simulink model "QAM_RX"  (R2018a)
settings: Solver=ode45  StartTime=0.0  StopTime=inf  RelTol=1e-3  EnableMultiTasking=on
values from neighbouring files (symbols this model uses):
  FrameTime = 0.000552    [qpsktxrx16.mat]
  qpsktxrx =     [qpsktxrx16.mat]
undefined symbols (not defined in the file or in its folder): dfilt, j
libraries: simulink x6, dspstat3 x6, dspobslib x6, dspsigops x5, commdigbbndam3 x4, commblkintrlv2 x4, commutil2 x4, commrflib2 x3, commblksprivate x2, dspspect3 x2, dspsrcs4 x2, commsink2 x2
(part 1 of 2)
settings Model: SimulationMode=accelerator  Creator=root  LastModifiedBy=n53s123
settings DataIOCC: LimitDataPoints=on  SaveFormat=Array
settings OptimizationCC: LifeSpan=inf
settings DebuggingCC: SolverPrmCheckMsg=warning  SFUnexpectedBacktrackingDiag=warning  SFNoUnconditionalDefaultTransitionDiag=warning  SFExecutionAtInitializationDiag=none
settings HardwareCC: ProdBitPerPointer=32  ProdBitPerSizeT=32  ProdBitPerPtrDiffT=32  ProdLargestAtomicFloat=None  ProdIntDivRoundTo=Undefined  ProdEndianess=Unspecified  ProdWordSize=32  ProdHWDeviceType=32-bit Generic
settings ModelReferenceCC: PropagateSignalLabelsOutOfModel=off
settings CodeAppCC: StateflowObjectComments=on
settings GRTTargetCC: TargetLangStandard=C89/C90 (ANSI)  GeneratePreprocessorConditionals=Disable all
settings ConfigComp: CovMetricSettings=dw  CovHtmlReporting=on  CovSaveCumulativeToWorkspaceVar=on  CovSaveSingleToWorkspaceVar=on  CovExternalEMLEnable=off  CovSFcnEnable=off

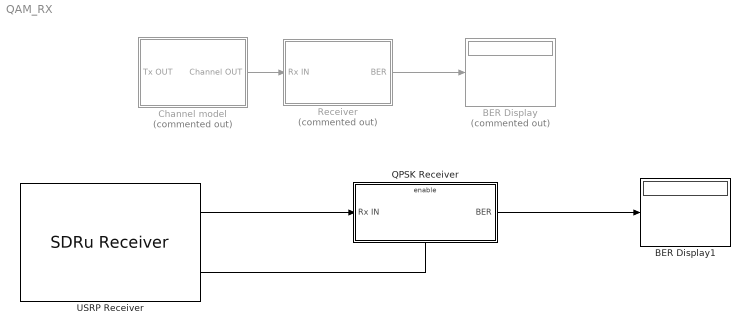
== system QAM_RX ==
  BER Display : Display  Commented=on
  BER Display1 : Display
  Channel model : Subsystem  Commented=on
  QPSK Receiver : Subsystem
      mask Display: disp('QAM Receiver')
  Receiver : Subsystem  Commented=on
      mask Display: disp('Receiver')
  USRP Receiver : commsdrhw_v2/SDRu Receiver  SourceLibraryInfo="This block requires <a href=\"http://www.mathworks.com/hardware-support/usrp.html\">Communications System Toolbox Support Package for USRP Radio</a>"  rxtx=rx  initializeIPAddress=0  devMap=0  USRP2_IP=192.168.10.2  USRP_IP_X300=192.168.10.2  USRP_IP_X310=192.168.10.2  USRP_serialNumB200=30B2ACA  USRP_serialNumB210=ECR04ZDBT  platform=N200/N210/USRP2  prevPlatform=N200/N210/USRP2  lastIPAddressPopup=192.168.10.2  USRP_ID=192.168.10.2  LastIPAddress=192.168.10.2  ChannelMapping=1  centerFrequencySrc=Dialog  centerFrequency=2.5e6  loOffsetSrc=Dialog  loOffset=0  gainSrc=Dialog  gain=0  PPSSource=Internal  clockSource=Internal  masterClkRateParam=100e6  masterClkRateB200=sdrqpskrx.MasterClockRate  masterClkRateB210=sdrqpskrx.MasterClockRate  masterClkRateX300=200e6  masterClkRateX310=200e6  masterClkRate=100e6  decimInterpSrc=Dialog  decimInterp=512  USRP2_IP_NUM=[49 57 50 46 49 54 56 46 49 48 46 50]  TransportDataType=int16  overrunUnderrunPort=off  sampleTime=1/qpsktxrx.DataLength*FrameTime  outputDatatype=double  frameLength=276  HOST_DATA_PORT=0  HOST_CONTROL_PORT=0  USRP2_DATA_PORT=0  USRP2_CONTROL_PORT=0  bufferMode=Continuous streaming  EnableBurstMode=off  NumFramesInBurst=100
      settings: SourceProductName=Communications System Toolbox Support Package for USRP(R) Radio  SourceProductBaseCode=USRP
  wires:
  Receiver/1(BER) -> BER Display/1
  USRP Receiver/1 -> QPSK Receiver/1(Rx IN)
  USRP Receiver/2 -> QPSK Receiver/Enable
  QPSK Receiver/1(BER) -> BER Display1/1
  Channel model/1(Channel OUT) -> Receiver/1(Rx IN)

== system QAM_RX/Channel model ==
  Tx OUT : Inport
  AWGN Channel : commchan3/AWGN Channel  InputProcessing=Columns as channels (frame based)  seed=67  noiseMode="Signal to noise ratio  (Eb/No)"  EbNodB=15  EsNodB=15  SNRdB=15  bitsPerSym=4  Ps=3/qpsktxrx.Upsampling  Tsym=qpsktxrx.Upsampling*qpsktxrx.Ts  variance=1
  Delay Generator : Subsystem
      mask Display: disp('Delay Generator')
  Delay Select : Constant  Value=2
  MATLAB Function : MATLAB Function  TreatAsAtomicUnit=on
  Phase/ Frequency Offset : commrflib2/Phase// Frequency Offset  phaseOffset=10  freqPort=off  freqOffset=1000
      settings: SourceProductName=Communications System Toolbox
  Variable Fractional Delay : dspsigops/Variable Fractional Delay  mode=OBSOLETE  modeActive=Linear  dmax=qpsktxrx.FrameSize*qpsktxrx.Upsampling  InputProcessing=Columns as channels (frame based)  L=4  FarrowL=4  R=10  alpha=1  ic=0  fallbackFIR=Clip to the minimum value necessary for centered kernel  fallbackFarrow=Clip to the minimum value necessary for centered kernel  noDFT=off  roundingMode=Zero  overflowMode=off
      settings: SourceProductName=DSP System Toolbox  SourceProductBaseCode=DS
  Channel OUT : Outport
  wires:
  Delay Select/1 -> Delay Generator/1(Delay Select)
  MATLAB Function/1(y) -> AWGN Channel/1
  Tx OUT/1 -> Phase/ Frequency Offset/1
  AWGN Channel/1 -> Channel OUT/1
  Phase/ Frequency Offset/1 -> Variable Fractional Delay/1
  Variable Fractional Delay/1 -> MATLAB Function/1(u)
  Delay Generator/1(Delay) -> Variable Fractional Delay/2

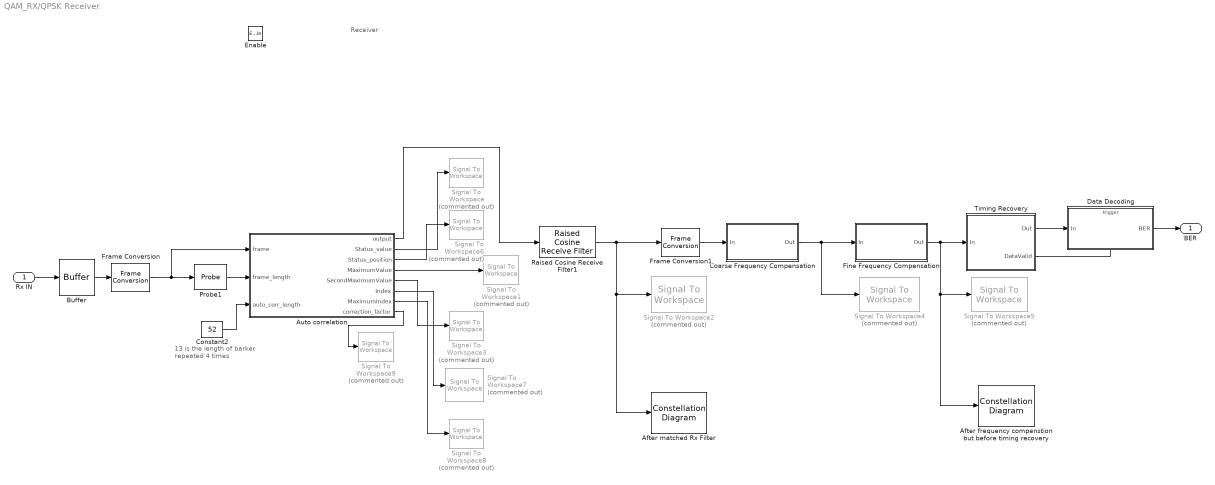
== system QAM_RX/QPSK Receiver ==
  note: Receiver
  note: 13 is the length of barker
      | repeated 4 times
  Rx IN : Inport
  Enable : EnablePort  PropagateVarSize=During execution
  After frequency compenstion but before timing recovery : ConstellationDiagram  Tag=ScatterPlot
  After matched Rx Filter : ConstellationDiagram  Tag=ScatterPlot
  Auto correlation : MATLAB Function  TreatAsAtomicUnit=on
  Buffer : Buffer  N=qpsktxrx.FrameSize*qpsktxrx.Upsampling*qpsktxrx.RxBufferedFrames
  Coarse Frequency Compensation : Subsystem
      mask Display: disp('Coarse Frequency\nCompensation');
  Constant2 : Constant  Value=52  VectorParams1D=off  OutDataTypeStr=Inherit: Inherit via back propagation  FramePeriod=2
  Data Decoding : Subsystem
      mask Display: disp('Data Decoding');
  Fine Frequency Compensation : Subsystem
      mask Display: disp('Fine Frequency\nCompensation')
  Frame Conversion : FrameConversion  OutFrame=Sample-based
  Frame Conversion1 : FrameConversion  OutFrame=Sample-based
  Probe1 : Probe  ProbeSampleTime=off  ProbeComplexSignal=off
  Raised Cosine Receive Filter1 : commfilt2/Raised Cosine Receive Filter  filtType=Square root  R=0.5  filtSpan=qpsktxrx.RaisedCosineFilterSpan  N=qpsktxrx.Upsampling  downFactor=qpsktxrx.Downsampling  downOffset=0  filterGain=1  InputProcessing=Columns as channels (frame based)  RateOptions=Enforce single-rate processing  framing=Mute  checkCoeff=off  variableName=rcRxFilt1  currentFiltSpan=qpsktxrx.RaisedCosineFilterSpan  D=(qpsktxrx.RaisedCosineFilterSpan)/2  inputOffset=0  sampMode=Mute  saveAsFlag=0  rateMode=Downsampling  checkGain=Normalized  launchFVT=off  roundingMode=Floor  overflowMode=off  coeffDataTypeStr=Inherit: Same word length as input  coeffMin=[]  coeffMax=[]  coeffLastDataTypeStr=Inherit: Same word length as input  accumDataTypeStr=Inherit: Same as product output  accumLastDataTypeStr=Inherit: Same as product output  outputDataTypeStr=Inherit: Same as accumulator  outputMin=[]  outputMax=[]  outputLastDataTypeStr=Inherit: Same as accumulator
  Signal To Workspace : SignalToWorkspace  Commented=on  VariableName=Status_value1
      settings: CopyFcn=dspblkcopystw(gcbh);
  Signal To Workspace1 : SignalToWorkspace  Commented=on  VariableName=MaxValue1
      settings: CopyFcn=dspblkcopystw(gcbh);
  Signal To Workspace2 : SignalToWorkspace  Commented=on  VariableName=data_Read
      settings: CopyFcn=dspblkcopystw(gcbh);
  Signal To Workspace3 : SignalToWorkspace  Commented=on  VariableName=SecondMaxValue1
      settings: CopyFcn=dspblkcopystw(gcbh);
  Signal To Workspace4 : SignalToWorkspace  Commented=on  VariableName=data_Read1
      settings: CopyFcn=dspblkcopystw(gcbh);
  Signal To Workspace5 : SignalToWorkspace  Commented=on  VariableName=data_Read5
      settings: CopyFcn=dspblkcopystw(gcbh);
  Signal To Workspace6 : SignalToWorkspace  Commented=on  VariableName=Status_position1
      settings: CopyFcn=dspblkcopystw(gcbh);
  Signal To Workspace7 : SignalToWorkspace  Commented=on  VariableName=SecondMaxIndex1
      settings: CopyFcn=dspblkcopystw(gcbh);
  Signal To Workspace8 : SignalToWorkspace  Commented=on  VariableName=MaxIndex1
      settings: CopyFcn=dspblkcopystw(gcbh);
  Signal To Workspace9 : SignalToWorkspace  Commented=on  VariableName=correection1
      settings: CopyFcn=dspblkcopystw(gcbh);
  Timing Recovery : Subsystem
      mask Display:
      | disp('Timing\nRecovery');
      | port_label('output',1,'DataOut');
      | port_label('output',2,'DataValid');
  BER : Outport
  wires:
  Auto correlation/5(SecondMaximumValue) -> Signal To Workspace3/1
  Probe1/1 -> Auto correlation/2(frame_length)
  Auto correlation/8(correction_factor) -> Signal To Workspace9/1
  Auto correlation/1(output) -> Raised Cosine Receive Filter1/1
  Frame Conversion1/1 -> Coarse Frequency Compensation/1(In)
  Fine Frequency Compensation/1(Out) -> After frequency compenstion but before timing recovery/1, Signal To Workspace5/1, Timing Recovery/1(In)
  Auto correlation/6(Index) -> Signal To Workspace7/1
  Frame Conversion/1 -> Auto correlation/1(frame), Probe1/1
  Auto correlation/7(MaximumIndex) -> Signal To Workspace8/1
  Constant2/1 -> Auto correlation/3(auto_corr_length)
  Auto correlation/4(MaximumValue) -> Signal To Workspace1/1
  Auto correlation/2(Status_value) -> Signal To Workspace/1
  Data Decoding/1(BER) -> BER/1
  Timing Recovery/2(DataValid) -> Data Decoding/Trigger
  Coarse Frequency Compensation/1(Out) -> Signal To Workspace4/1, Fine Frequency Compensation/1(In)
  Raised Cosine Receive Filter1/1 -> After matched Rx Filter/1, Signal To Workspace2/1, Frame Conversion1/1
  Buffer/1 -> Frame Conversion/1
  Timing Recovery/1(Out) -> Data Decoding/1(In)
  Rx IN/1 -> Buffer/1
  Auto correlation/3(Status_position) -> Signal To Workspace6/1

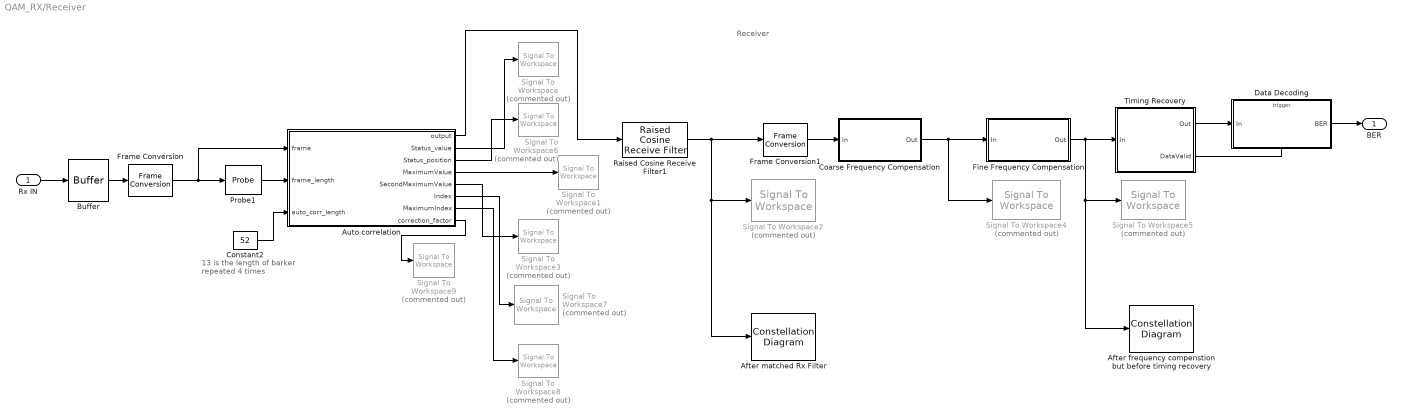
== system QAM_RX/Receiver ==
  note: 13 is the length of barker
      | repeated 4 times
  note: Receiver
  Rx IN : Inport
  After frequency compenstion but before timing recovery : ConstellationDiagram  Tag=ScatterPlot
  After matched Rx Filter : ConstellationDiagram  Tag=ScatterPlot
  Auto correlation : MATLAB Function  TreatAsAtomicUnit=on
  Buffer : Buffer  N=qpsktxrx.FrameSize*qpsktxrx.Upsampling*qpsktxrx.RxBufferedFrames
  Coarse Frequency Compensation : Subsystem
      mask Display: disp('Coarse Frequency\nCompensation');
  Constant2 : Constant  Value=52  VectorParams1D=off  OutDataTypeStr=Inherit: Inherit via back propagation  FramePeriod=2
  Data Decoding : Subsystem
      mask Display: disp('Data Decoding');
  Fine Frequency Compensation : Subsystem
      mask Display: disp('Fine Frequency\nCompensation')
  Frame Conversion : FrameConversion  OutFrame=Sample-based
  Frame Conversion1 : FrameConversion  OutFrame=Sample-based
  Probe1 : Probe  ProbeSampleTime=off  ProbeComplexSignal=off
  Raised Cosine Receive Filter1 : commfilt2/Raised Cosine Receive Filter  filtType=Square root  R=0.5  filtSpan=qpsktxrx.RaisedCosineFilterSpan  N=qpsktxrx.Upsampling  downFactor=qpsktxrx.Downsampling  downOffset=0  filterGain=1  InputProcessing=Columns as channels (frame based)  RateOptions=Enforce single-rate processing  framing=Mute  checkCoeff=off  variableName=rcRxFilt1  currentFiltSpan=qpsktxrx.RaisedCosineFilterSpan  D=(qpsktxrx.RaisedCosineFilterSpan)/2  inputOffset=0  sampMode=Mute  saveAsFlag=0  rateMode=Downsampling  checkGain=Normalized  launchFVT=off  roundingMode=Floor  overflowMode=off  coeffDataTypeStr=Inherit: Same word length as input  coeffMin=[]  coeffMax=[]  coeffLastDataTypeStr=Inherit: Same word length as input  accumDataTypeStr=Inherit: Same as product output  accumLastDataTypeStr=Inherit: Same as product output  outputDataTypeStr=Inherit: Same as accumulator  outputMin=[]  outputMax=[]  outputLastDataTypeStr=Inherit: Same as accumulator
  Signal To Workspace : SignalToWorkspace  Commented=on  VariableName=Status_value
      settings: CopyFcn=dspblkcopystw(gcbh);
  Signal To Workspace1 : SignalToWorkspace  Commented=on  VariableName=MaxValue
      settings: CopyFcn=dspblkcopystw(gcbh);
  Signal To Workspace2 : SignalToWorkspace  Commented=on  VariableName=data_Read2
      settings: CopyFcn=dspblkcopystw(gcbh);
  Signal To Workspace3 : SignalToWorkspace  Commented=on  VariableName=SecondMaxValue
      settings: CopyFcn=dspblkcopystw(gcbh);
  Signal To Workspace4 : SignalToWorkspace  Commented=on  VariableName=data_Read3
      settings: CopyFcn=dspblkcopystw(gcbh);
  Signal To Workspace5 : SignalToWorkspace  Commented=on  VariableName=data_Read4
      settings: CopyFcn=dspblkcopystw(gcbh);
  Signal To Workspace6 : SignalToWorkspace  Commented=on  VariableName=Status_position
      settings: CopyFcn=dspblkcopystw(gcbh);
  Signal To Workspace7 : SignalToWorkspace  Commented=on  VariableName=SecondMaxIndex
      settings: CopyFcn=dspblkcopystw(gcbh);
  Signal To Workspace8 : SignalToWorkspace  Commented=on  VariableName=MaxIndex
      settings: CopyFcn=dspblkcopystw(gcbh);
  Signal To Workspace9 : SignalToWorkspace  Commented=on  VariableName=correection
      settings: CopyFcn=dspblkcopystw(gcbh);
  Timing Recovery : Subsystem
      mask Display:
      | disp('Timing\nRecovery');
      | port_label('output',1,'DataOut');
      | port_label('output',2,'DataValid');
  BER : Outport
  wires:
  Timing Recovery/1(Out) -> Data Decoding/1(In)
  Data Decoding/1(BER) -> BER/1
  Timing Recovery/2(DataValid) -> Data Decoding/Trigger
  Rx IN/1 -> Buffer/1
  Buffer/1 -> Frame Conversion/1
  Constant2/1 -> Auto correlation/3(auto_corr_length)
  Auto correlation/2(Status_value) -> Signal To Workspace/1
  Auto correlation/4(MaximumValue) -> Signal To Workspace1/1
  Auto correlation/5(SecondMaximumValue) -> Signal To Workspace3/1
  Auto correlation/3(Status_position) -> Signal To Workspace6/1
  Auto correlation/7(MaximumIndex) -> Signal To Workspace8/1
  Auto correlation/6(Index) -> Signal To Workspace7/1
  Probe1/1 -> Auto correlation/2(frame_length)
  Frame Conversion/1 -> Auto correlation/1(frame), Probe1/1
  Auto correlation/8(correction_factor) -> Signal To Workspace9/1
  Auto correlation/1(output) -> Raised Cosine Receive Filter1/1
  Frame Conversion1/1 -> Coarse Frequency Compensation/1(In)
  Fine Frequency Compensation/1(Out) -> After frequency compenstion but before timing recovery/1, Signal To Workspace5/1, Timing Recovery/1(In)
  Raised Cosine Receive Filter1/1 -> After matched Rx Filter/1, Signal To Workspace2/1, Frame Conversion1/1
  Coarse Frequency Compensation/1(Out) -> Signal To Workspace4/1, Fine Frequency Compensation/1(In)

== system QAM_RX/Channel model/Delay Generator ==
  Delay Select : Inport
  Multiport Switch : MultiPortSwitch  Inputs=2  OutDataTypeStr=double
  Repeating Sequence Stair : simulink/Sources/Repeating Sequence Stair  OutValues="[0        0.05         0.1        0.15         0.2        0.25         0.3        0.35         0.4        0.45         0.5        0.55         0.6        0.65         0.7        0.75         0.8        0.85         0.9        0.95           1        1.05         1.1        1.15         1.2        1.25         1.3        1.35         1.4        1.45         1.5        1.55         1.6        1.65         1.7        1.75         1.8        1.85         1.9        1.95           2        2.05         2.1        2.15         2.2        2.25         2.3        2.35         2.4        2.45         2.5        2.55         2.6        2.65         2.7        2.75         2.8        2.85         2.9        2.95           3        3.05         3.1        3.15         3.2        3.25         3.3        3.35         3.4        3.45         3.5        3.55         3.6        3.65         3.7        3.75         3.8        3.85         3.9        3.95           4        4.05         4.1        4.15         4.2        4.25         4.3        4.35         4.4        4.45         4.5        4.55         4.6        4.65         4.7        4.75         4.8        4.85         4.9        4.95           5        5.05         5.1        5.15         5.2        5.25         5.3        5.35         5.4        5.45         5.5        5.55         5.6        5.65         5.7        5.75         5.8        5.85         5.9        5.95           6        6.05         6.1        6.15         6.2        6.25         6.3        6.35         6.4        6.45         6.5        6.55         6.6        6.65         6.7        6.75         6.8        6.85         6.9        6.95           7        7.05         7.1        7.15         7.2        7.25         7.3        7.35         7.4        7.45         7.5        7.55         7.6        7.65         7.7        7.75         7.8        7.85         7.9        7.95           8        7.95         7.9        7.85         7.8        7.75         7.7        7.65         7.6        7.55         7.5        7.45         7.4        7.35         7.3        7.25         7.2        7.15         7.1        7.05           7        6.95         6.9        6.85         6.8        6.75         6.7        6.65         6.6        6.55         6.5        6.45         6.4        6.35         6.3        6.25         6.2        6.15         6.1        6.05           6        5.95         5.9        5.85         5.8        5.75         5.7        5.65         5.6        5.55         5.5        5.45         5.4        5.35         5.3        5.25         5.2        5.15         5.1        5.05           5        4.95         4.9        4.85         4.8        4.75         4.7        4.65         4.6        4.55         4.5        4.45         4.4        4.35         4.3        4.25         4.2        4.15         4.1        4.05           4        3.95         3.9        3.85         3.8        3.75         3.7        3.65         3.6        3.55         3.5        3.45         3.4        3.35         3.3        3.25         3.2        3.15         3.1        3.05           3        2.95         2.9        2.85         2.8        2.75         2.7        2.65         2.6        2.55         2.5        2.45         2.4        2.35         2.3        2.25         2.2        2.15         2.1        2.05           2        1.95         1.9        1.85         1.8        1.75         1.7        1.65         1.6        1.55         1.5        1.45         1.4        1.35         1.3        1.25         1.2        1.15         1.1        1.05           1        0.95         0.9        0.85         0.8        0.75         0.7        0.65         0.6        0.55         0.5        0.45         0.4        0.35         0.3        0.25         0.2        0.15         0.1        0.05]"  tsamp=qpsktxrx.FrameSize*qpsktxrx.Upsampling*qpsktxrx.Ts  OutMin=[]  OutMax=[]  OutDataTypeStr=double  OutputDataTypeScalingMode=double  OutDataType=fixdt(0,8)  ConRadixGroup=Best Precision: Vector-wise  OutScaling=2^-12
  mVariableRamp : Subsystem
  Delay : Outport
  wires:
  Delay Select/1 -> Multiport Switch/1
  Repeating Sequence Stair/1 -> Multiport Switch/3
  mVariableRamp/1(Out) -> Multiport Switch/2
  Multiport Switch/1 -> Delay/1

== system QAM_RX/QPSK Receiver/Coarse Frequency Compensation ==
  In : Inport
  Compensate for Frequency Offset : commrflib2/Phase// Frequency Offset  phaseOffset=0  freqPort=on  freqOffset=100
      settings: SourceProductName=Communications System Toolbox
  Estimated Frequency Offset : Scope
  Find Frequency Offset : Subsystem
  Gain : Gain  Gain=-1
  Signal To Workspace1 : SignalToWorkspace  Commented=on  VariableName=Freq_corrected
      settings: CopyFcn=dspblkcopystw(gcbh);  Save2DSignal=3-D array (concatenate along third dimension)
  Out : Outport
  wires:
  Find Frequency Offset/1(Freq Offset) -> Gain/1, Estimated Frequency Offset/1
  In/1 -> Compensate for Frequency Offset/1, Find Frequency Offset/1(In)
  Compensate for Frequency Offset/1 -> Signal To Workspace1/1, Out/1
  Gain/1 -> Compensate for Frequency Offset/2

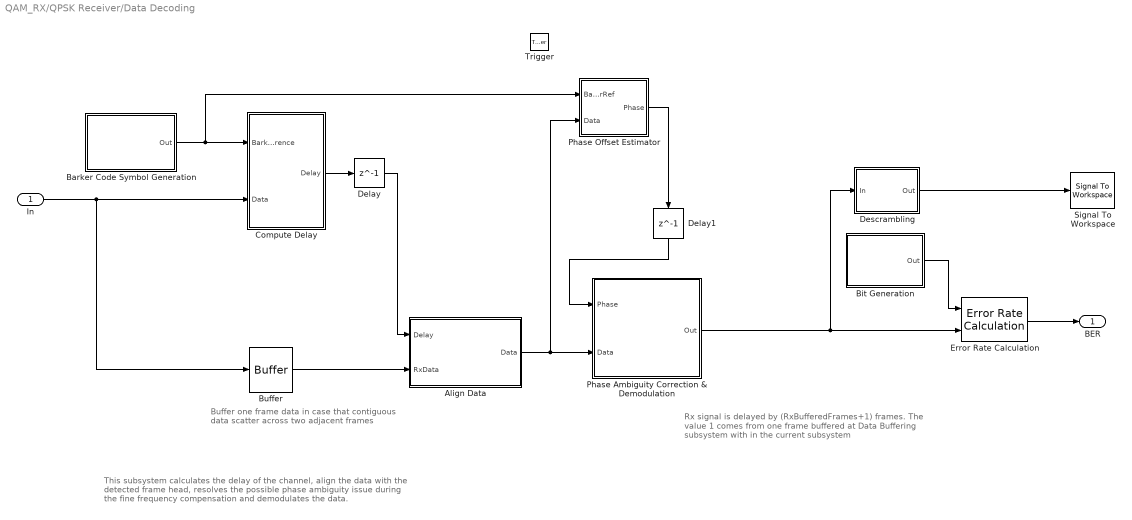
== system QAM_RX/QPSK Receiver/Data Decoding ==
  note: Buffer one frame data in case that contiguous
      | data scatter across two adjacent frames
  note: This subsystem calculates the delay of the channel, align the data with
      | the detected frame head, resolves the possible phase ambiguity issue
      | during the fine frequency compensation and demodulates the data.
  note: Rx signal is delayed by (RxBufferedFrames+1) frames.
      | The value 1 comes from one frame buffered at Data
      | Buffering subsystem with in the current subsystem
  In : Inport
  Trigger : TriggerPort  VariantControl=(inherit)  PortDimensions=1
  Align Data : MATLAB Function  TreatAsAtomicUnit=on
  "Barker Code Symbol Generation " : Subsystem
      mask Display: disp('Barker Code\nSymbol Generation')
  Bit Generation : Subsystem
      mask Display: disp('Bits Generation')
  Buffer : Buffer  N=qpsktxrx.FrameSize*2  V=qpsktxrx.FrameSize
  Compute Delay : Subsystem
      mask Display: disp('Compute\nDelay');
  Delay : Delay  DelayLength=1
  Delay1 : Delay  DelayLength=1
  Descrambling : Subsystem
      mask Display: disp('Descrambling');
  Error Rate Calculation : commsink2/Error Rate Calculation  N=(qpsktxrx.RxBufferedFrames+1)*qpsktxrx.FrameSize*log2(qpsktxrx.M)  st_delay=(qpsktxrx.RxBufferedFrames+1)*qpsktxrx.FrameSize*log2(qpsktxrx.M)  cp_mode=Entire frame  subframe=sdrqpskrx.BerMask  PMode=Port  WsName=ErrorVec  RsMode2=off  stop=off  numErr=100  maxBits=1e6
  Phase Ambiguity Correction & Demodulation : Subsystem
      mask Display: disp('Phase Ambiguity\nCorrection\n& Demodulation');
  Phase Offset Estimator : Subsystem
  Signal To Workspace : SignalToWorkspace  VariableName=RxData
      settings: CopyFcn=dspblkcopystw(gcbh);
  BER : Outport
  wires:
  Delay/1 -> Align Data/1(Delay)
  Buffer/1 -> Align Data/2(RxData)
  In/1 -> Compute Delay/2(Data), Buffer/1
  Compute Delay/1(Delay) -> Delay/1
  "Barker Code Symbol Generation "/1(Out) -> Compute Delay/1(Barker Reference), Phase Offset Estimator/1(BarkerRef)
  Align Data/1(Data) -> Phase Ambiguity Correction & Demodulation/2(Data), Phase Offset Estimator/2(Data)
  Phase Ambiguity Correction & Demodulation/1(Out) -> Descrambling/1(In), Error Rate Calculation/2
  Phase Offset Estimator/1(Phase) -> Delay1/1
  Delay1/1 -> Phase Ambiguity Correction & Demodulation/1(Phase)
  Descrambling/1(Out) -> Signal To Workspace/1
  Error Rate Calculation/1 -> BER/1
  Bit Generation/1(Out) -> Error Rate Calculation/1

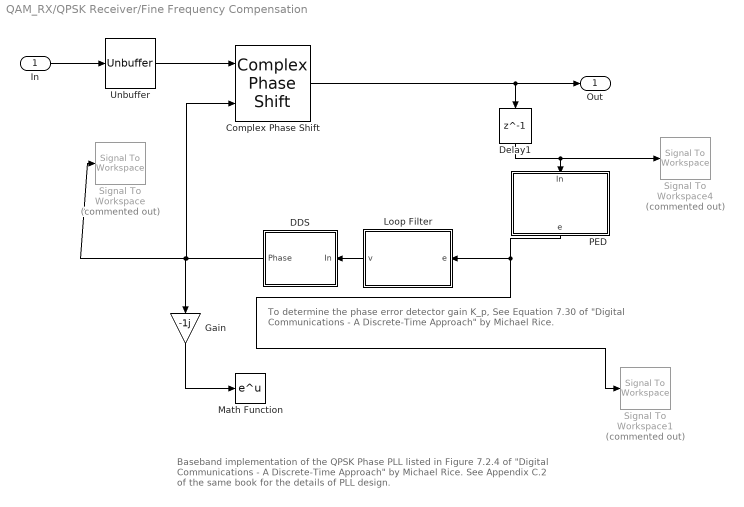
== system QAM_RX/QPSK Receiver/Fine Frequency Compensation ==
  note: To determine the phase error detector gain K_p, See Equation 7.30 of "Digital
      | Communications - A Discrete-Time Approach" by Michael Rice.
  note: Baseband implementation of the QPSK Phase PLL listed in Figure 7.2.4 of
      | "Digital Communications - A Discrete-Time Approach" by Michael Rice. See
      | Appendix C.2 of the same book for the details of PLL design.
  In : Inport
  Complex Phase Shift : commutil2/Complex Phase Shift
      settings: SourceProductName=Communications System Toolbox  SourceProductBaseCode=CM
  DDS : Subsystem
      mask Display: disp('DDS')
  Delay1 : Delay  DelayLength=1  InitialCondition=0  InputProcessing=Columns as channels (frame based)
  Gain : Gain  Gain=-1j
  Loop Filter : Subsystem  mask{BnTs=0.01, zeta=1, N=qpsktxrx.Upsampling/qpsktxrx.Downsampling, Kp=qpsktxrx.PhaseErrorDetectorGain, K0=qpsktxrx.PhaseRecoveryGain}
      mask prompts: BnTs "Normalized Loop Bandwidth"; zeta "Damping Factor"; N "Number of Samples/Symbol"; Kp "Phase Detector Gain (Kp)"; K0 "DDS Gain (K0)"
      mask init:
      | % See C.57 to C.61 in Michael Rice's "Digital Communications 
      | % - A Discrete-Time Approach" for details
      | theta = BnTs/(zeta+0.25/zeta)/N;
      | d = 1 + 2*zeta*theta + theta*theta;
      | K1 = 4*zeta*theta/d;
      | K2 = 4*theta*theta/d;
      | K1 = K1/(Kp*K0);
      | K2 = K2/(Kp*K0);
      mask Display: disp('Loop Filter')
  Math Function : Math  SaturateOnIntegerOverflow=on
  PED : MATLAB Function  TreatAsAtomicUnit=on
  Signal To Workspace : SignalToWorkspace  Commented=on  VariableName=phase_estimate
      settings: CopyFcn=dspblkcopystw(gcbh);  Save2DSignal=3-D array (concatenate along third dimension)
  Signal To Workspace1 : SignalToWorkspace  Commented=on  VariableName=PED
      settings: CopyFcn=dspblkcopystw(gcbh);  Save2DSignal=3-D array (concatenate along third dimension)
  Signal To Workspace4 : SignalToWorkspace  Commented=on  VariableName=before_PED
      settings: CopyFcn=dspblkcopystw(gcbh);  Save2DSignal=3-D array (concatenate along third dimension)
  Unbuffer : Unbuffer
  Out : Outport
  wires:
  Gain/1 -> Math Function/1
  PED/1(e) -> Loop Filter/1(e), Signal To Workspace1/1
  Loop Filter/1(v) -> DDS/1(In)
  In/1 -> Unbuffer/1
  Complex Phase Shift/1 -> Delay1/1, Out/1
  Unbuffer/1 -> Complex Phase Shift/1
  Delay1/1 -> Signal To Workspace4/1, PED/1(In)
  DDS/1(Phase) -> Signal To Workspace/1, Gain/1, Complex Phase Shift/2

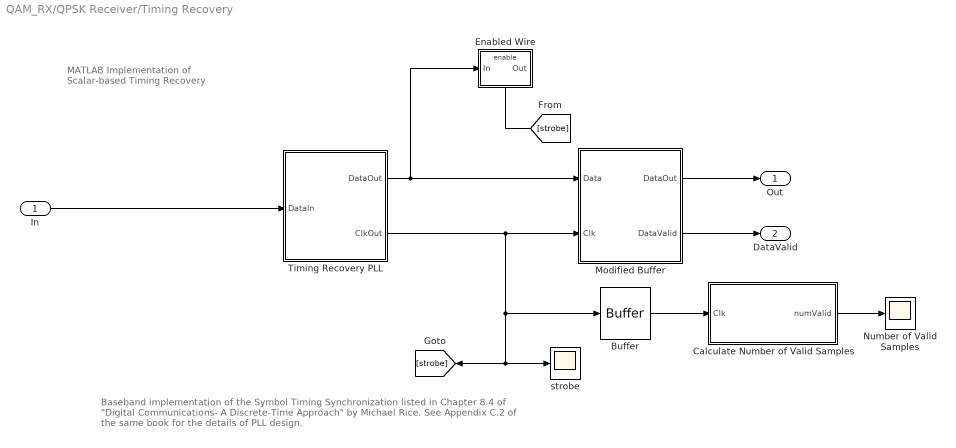
== system QAM_RX/QPSK Receiver/Timing Recovery ==
  note: Baseband implementation of the Symbol Timing Synchronization listed in Chapter 8.4
      | of "Digital Communications- A Discrete-Time Approach" by Michael Rice. See
      | Appendix C.2 of the same book for the details of PLL design.
  note: MATLAB Implementation
      | of Scalar-based Timing Recovery
  In : Inport
  Buffer : Buffer  N=qpsktxrx.FrameSize*qpsktxrx.Upsampling/qpsktxrx.Downsampling
  Calculate Number of Valid Samples : MATLAB Function  TreatAsAtomicUnit=on
  Enabled Wire : Subsystem  TreatAsAtomicUnit=on
  Modified Buffer : Subsystem  TreatAsAtomicUnit=on  mask(Input-Driven Buffer){bufSize=qpsktxrx.FrameSize}
      mask prompts: bufSize "Buffer size:"
      mask help: A modified buffer subsystem that is driven by the arrival of its input data; it produces a valid output data buffer whenever its buffer is full and sets its dataValid flag to 1. Otherwise, the data at its dataOut port is not valid and its dataValid flag is set to 0.
      mask Display: disp('Modified Buffer')
  Number of Valid Samples : Scope
  Timing Recovery PLL : Subsystem
      mask Display:
      | disp('Timing Recovery\nPLL')
      | port_label('input',1,'In')
      | port_label('output',1,'DataOut')
      | port_label('output',2,'Clk')
  strobe : Scope
  Out : Outport
  DataValid : Outport  Port=2
  wires:
  Timing Recovery PLL/2(ClkOut) -> [strobe], strobe/1, Buffer/1, Modified Buffer/2(Clk)
  Timing Recovery PLL/1(DataOut) -> Enabled Wire/1(In), Modified Buffer/1(Data)
  Calculate Number of Valid Samples/1(numValid) -> Number of Valid Samples/1
  [strobe] -> Enabled Wire/Enable
  In/1 -> Timing Recovery PLL/1(DataIn)
  Modified Buffer/1(DataOut) -> Out/1
  Modified Buffer/2(DataValid) -> DataValid/1
  Buffer/1 -> Calculate Number of Valid Samples/1(Clk)

== system QAM_RX/Receiver/Coarse Frequency Compensation ==
  In : Inport
  Compensate for Frequency Offset : commrflib2/Phase// Frequency Offset  phaseOffset=0  freqPort=on  freqOffset=100
      settings: SourceProductName=Communications System Toolbox
  Estimated Frequency Offset : Scope
  Find Frequency Offset : Subsystem
  Gain : Gain  Gain=-1
  Signal To Workspace1 : SignalToWorkspace  Commented=on  VariableName=Freq_corrected
      settings: CopyFcn=dspblkcopystw(gcbh);  Save2DSignal=3-D array (concatenate along third dimension)
  Out : Outport
  wires:
  Find Frequency Offset/1(Freq Offset) -> Gain/1, Estimated Frequency Offset/1
  In/1 -> Compensate for Frequency Offset/1, Find Frequency Offset/1(In)
  Compensate for Frequency Offset/1 -> Signal To Workspace1/1, Out/1
  Gain/1 -> Compensate for Frequency Offset/2

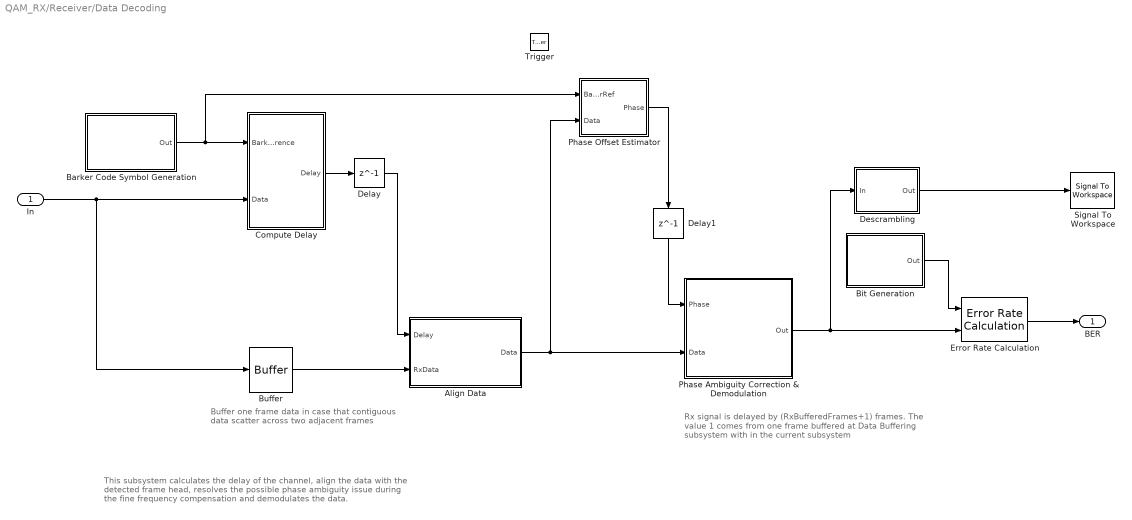
== system QAM_RX/Receiver/Data Decoding ==
  note: Buffer one frame data in case that contiguous
      | data scatter across two adjacent frames
  note: This subsystem calculates the delay of the channel, align the data with
      | the detected frame head, resolves the possible phase ambiguity issue
      | during the fine frequency compensation and demodulates the data.
  note: Rx signal is delayed by (RxBufferedFrames+1) frames.
      | The value 1 comes from one frame buffered at Data
      | Buffering subsystem with in the current subsystem
  In : Inport
  Trigger : TriggerPort  VariantControl=(inherit)  PortDimensions=1
  Align Data : MATLAB Function  TreatAsAtomicUnit=on
  "Barker Code Symbol Generation " : Subsystem
      mask Display: disp('Barker Code\nSymbol Generation')
  Bit Generation : Subsystem
      mask Display: disp('Bits Generation')
  Buffer : Buffer  N=qpsktxrx.FrameSize*2  V=qpsktxrx.FrameSize
  Compute Delay : Subsystem
      mask Display: disp('Compute\nDelay');
  Delay : Delay  DelayLength=1
  Delay1 : Delay  DelayLength=1
  Descrambling : Subsystem
      mask Display: disp('Descrambling');
  Error Rate Calculation : commsink2/Error Rate Calculation  N=(qpsktxrx.RxBufferedFrames+1)*qpsktxrx.FrameSize*log2(qpsktxrx.M)  st_delay=(qpsktxrx.RxBufferedFrames+1)*qpsktxrx.FrameSize*log2(qpsktxrx.M)  cp_mode=Entire frame  subframe=[]  PMode=Port  WsName=ErrorVec  RsMode2=off  stop=off  numErr=100  maxBits=1e6
  Phase Ambiguity Correction & Demodulation : Subsystem
      mask Display: disp('Phase Ambiguity\nCorrection\n& Demodulation');
  Phase Offset Estimator : Subsystem
  Signal To Workspace : SignalToWorkspace  VariableName=RxData
      settings: CopyFcn=dspblkcopystw(gcbh);
  BER : Outport
  wires:
  Delay/1 -> Align Data/1(Delay)
  Buffer/1 -> Align Data/2(RxData)
  In/1 -> Compute Delay/2(Data), Buffer/1
  Compute Delay/1(Delay) -> Delay/1
  "Barker Code Symbol Generation "/1(Out) -> Compute Delay/1(Barker Reference), Phase Offset Estimator/1(BarkerRef)
  Align Data/1(Data) -> Phase Ambiguity Correction & Demodulation/2(Data), Phase Offset Estimator/2(Data)
  Phase Ambiguity Correction & Demodulation/1(Out) -> Descrambling/1(In), Error Rate Calculation/2
  Phase Offset Estimator/1(Phase) -> Delay1/1
  Delay1/1 -> Phase Ambiguity Correction & Demodulation/1(Phase)
  Descrambling/1(Out) -> Signal To Workspace/1
  Error Rate Calculation/1 -> BER/1
  Bit Generation/1(Out) -> Error Rate Calculation/1

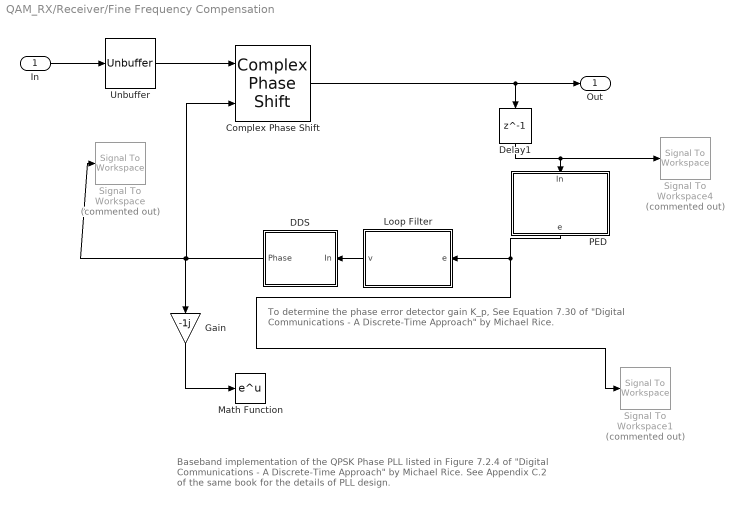
== system QAM_RX/Receiver/Fine Frequency Compensation ==
  note: To determine the phase error detector gain K_p, See Equation 7.30 of "Digital
      | Communications - A Discrete-Time Approach" by Michael Rice.
  note: Baseband implementation of the QPSK Phase PLL listed in Figure 7.2.4 of
      | "Digital Communications - A Discrete-Time Approach" by Michael Rice. See
      | Appendix C.2 of the same book for the details of PLL design.
  In : Inport
  Complex Phase Shift : commutil2/Complex Phase Shift
      settings: SourceProductName=Communications System Toolbox  SourceProductBaseCode=CM
  DDS : Subsystem
      mask Display: disp('DDS')
  Delay1 : Delay  DelayLength=1  InitialCondition=0  InputProcessing=Columns as channels (frame based)
  Gain : Gain  Gain=-1j
  Loop Filter : Subsystem  mask{BnTs=0.01, zeta=1, N=qpsktxrx.Upsampling/qpsktxrx.Downsampling, Kp=qpsktxrx.PhaseErrorDetectorGain, K0=qpsktxrx.PhaseRecoveryGain}
      mask prompts: BnTs "Normalized Loop Bandwidth"; zeta "Damping Factor"; N "Number of Samples/Symbol"; Kp "Phase Detector Gain (Kp)"; K0 "DDS Gain (K0)"
      mask init: same as QAM_RX/QPSK Receiver/Fine Frequency Compensation/Loop Filter
      mask Display: disp('Loop Filter')
  Math Function : Math  SaturateOnIntegerOverflow=on
  PED : MATLAB Function  TreatAsAtomicUnit=on
  Signal To Workspace : SignalToWorkspace  Commented=on  VariableName=phase_estimate
      settings: CopyFcn=dspblkcopystw(gcbh);  Save2DSignal=3-D array (concatenate along third dimension)
  Signal To Workspace1 : SignalToWorkspace  Commented=on  VariableName=PED
      settings: CopyFcn=dspblkcopystw(gcbh);  Save2DSignal=3-D array (concatenate along third dimension)
  Signal To Workspace4 : SignalToWorkspace  Commented=on  VariableName=before_PED
      settings: CopyFcn=dspblkcopystw(gcbh);  Save2DSignal=3-D array (concatenate along third dimension)
  Unbuffer : Unbuffer
  Out : Outport
  wires:
  Gain/1 -> Math Function/1
  PED/1(e) -> Loop Filter/1(e), Signal To Workspace1/1
  Loop Filter/1(v) -> DDS/1(In)
  In/1 -> Unbuffer/1
  Complex Phase Shift/1 -> Delay1/1, Out/1
  Unbuffer/1 -> Complex Phase Shift/1
  Delay1/1 -> Signal To Workspace4/1, PED/1(In)
  DDS/1(Phase) -> Signal To Workspace/1, Gain/1, Complex Phase Shift/2

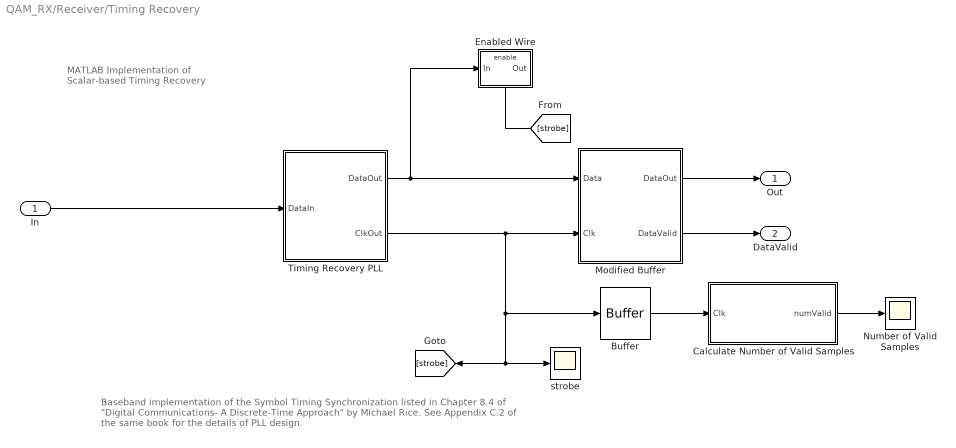
== system QAM_RX/Receiver/Timing Recovery ==
  note: Baseband implementation of the Symbol Timing Synchronization listed in Chapter 8.4
      | of "Digital Communications- A Discrete-Time Approach" by Michael Rice. See
      | Appendix C.2 of the same book for the details of PLL design.
  note: MATLAB Implementation
      | of Scalar-based Timing Recovery
  In : Inport
  Buffer : Buffer  N=qpsktxrx.FrameSize*qpsktxrx.Upsampling/qpsktxrx.Downsampling
  Calculate Number of Valid Samples : MATLAB Function  TreatAsAtomicUnit=on
  Enabled Wire : Subsystem  TreatAsAtomicUnit=on
  Modified Buffer : Subsystem  TreatAsAtomicUnit=on  mask(Input-Driven Buffer){bufSize=qpsktxrx.FrameSize}
      mask prompts: bufSize "Buffer size:"
      mask help: A modified buffer subsystem that is driven by the arrival of its input data; it produces a valid output data buffer whenever its buffer is full and sets its dataValid flag to 1. Otherwise, the data at its dataOut port is not valid and its dataValid flag is set to 0.
      mask Display: disp('Modified Buffer')
  Number of Valid Samples : Scope
  Timing Recovery PLL : Subsystem
      mask Display:
      | disp('Timing Recovery\nPLL')
      | port_label('input',1,'In')
      | port_label('output',1,'DataOut')
      | port_label('output',2,'Clk')
  strobe : Scope
  Out : Outport
  DataValid : Outport  Port=2
  wires:
  Timing Recovery PLL/2(ClkOut) -> [strobe], strobe/1, Buffer/1, Modified Buffer/2(Clk)
  Timing Recovery PLL/1(DataOut) -> Enabled Wire/1(In), Modified Buffer/1(Data)
  Calculate Number of Valid Samples/1(numValid) -> Number of Valid Samples/1
  [strobe] -> Enabled Wire/Enable
  In/1 -> Timing Recovery PLL/1(DataIn)
  Modified Buffer/1(DataOut) -> Out/1
  Modified Buffer/2(DataValid) -> DataValid/1
  Buffer/1 -> Calculate Number of Valid Samples/1(Clk)

== system QAM_RX/Channel model/Delay Generator/mVariableRamp ==
  Add : Sum
  Constant1 : Constant  Value=(qpsktxrx.FrameSize-qpsktxrx.RaisedCosineFilterSpan)*qpsktxrx.Upsampling
  Counter Free-Running : simulink/Sources/Counter Free-Running  NumBits=64  tsamp=qpsktxrx.FrameSize*qpsktxrx.Upsampling*qpsktxrx.Ts
  Divide : Product  Inputs=**
  MinMax : MinMax  Inputs=2
  Start : Constant  Value=0.1
  Step : Constant  Value=0.05
  Out : Outport
  wires:
  Counter Free-Running/1 -> Divide/1
  Step/1 -> Divide/2
  Divide/1 -> Add/1
  Start/1 -> Add/2
  Add/1 -> MinMax/1
  MinMax/1 -> Out/1
  Constant1/1 -> MinMax/2

== system QAM_RX/QPSK Receiver/Coarse Frequency Compensation/Find Frequency Offset ==
  note: This subsystem does the following:
      | 1.  Creates a tone at M*Foffset, where M is the modulation order of the signal
      | 2.  Finds the index of the maximum amplitude across the frequency band
      | 3.  Converts the index to the frequency offset according to
      | Foffset = IndexofMaxAmplitude * FrameSize / (FFTLength * M * FrameSampleTime)
  In : Inport
  Alphabet size : Constant  Value=4  OutDataTypeStr=Inherit: Inherit via back propagation
  Complex Power : commblksprivate/Complex Power
      settings: SourceProductName=Communications System Toolbox  SourceProductBaseCode=CM
  Find Frequency Offset : MATLAB Function  TreatAsAtomicUnit=on
  Periodogram : dspspect3/Periodogram  measurement=Power spectral density  wintype=Hamming  Rs=50  beta=5  winsamp=Symmetric  FFTImplementation=Auto  inheritFFT=off  fftsize=2048  navg=2  inheritTs=on  Ts=1
      settings: SourceProductName=DSP System Toolbox  SourceProductBaseCode=DS
  Probe : Probe  ProbeComplexSignal=off
  Signal To Workspace : SignalToWorkspace  Commented=on  VariableName=width
      settings: CopyFcn=dspblkcopystw(gcbh);  Save2DSignal=3-D array (concatenate along third dimension)
  Freq Offset : Outport
  wires:
  Periodogram/1 -> Find Frequency Offset/3(FFTSig)
  Alphabet size/1 -> Complex Power/2
  In/1 -> Complex Power/1
  Probe/1 -> Find Frequency Offset/1(N)
  Probe/2 -> Find Frequency Offset/2(Tf)
  Find Frequency Offset/1(FreqOffset) -> Signal To Workspace/1, Freq Offset/1
  Complex Power/1 -> Probe/1, Periodogram/1

== system QAM_RX/QPSK Receiver/Data Decoding/Barker Code Symbol Generation  ==
  note: Regenerate a QPSK-modulated unipolar Barker code sequence
      | to be compared with the received data
  Constant Barker Code : Constant  Value=|  VectorParams1D=off  OutDataTypeStr=double
      | [+1 +1 +1 +1 +1 -1 -1 +1 +1 -1 +1 -1 +1
      | ].' > 0
  Matrix Concatenate : Concatenate  Mode=Multidimensional array
  Rectangular QAM Modulator Baseband : commdigbbndam3/Rectangular QAM Modulator Baseband  M=16  InType=Bit  Enc=Gray  Mapping=[0:15]  PowType=Min. distance between symbols  MinDist=2  AvgPow=1  PeakPow=1  Ph=0  outDtype=double  outWordLen=16  outUDDataType=sfix(16)  outFracLenMode=Best precision  outFracLen=15  outDataTypeStr=double  outLastDataTypeStr=double
  Repeat : dspsigops/Repeat  N=4  InputProcessing=Columns as channels (frame based)  RateOptions=Enforce single-rate processing  ic=0  mode=Unused parameter value
      settings: SourceProductName=DSP System Toolbox
  Out : Outport
  wires:
  Constant Barker Code/1 -> Repeat/1
  Repeat/1 -> Rectangular QAM Modulator Baseband/1
  Rectangular QAM Modulator Baseband/1 -> Matrix Concatenate/2, Matrix Concatenate/1
  Matrix Concatenate/1 -> Out/1

== system QAM_RX/QPSK Receiver/Data Decoding/Bit Generation ==
  note: Each data frame contains 26 bits header (For Sync Purpose) and 174 bits data bits,
      | first 105 bits contain "Hello world ###" message. Scrambler is there to improve data
      | transition density and frequency offset estimation.
  Barker Code SS : Subsystem
      mask Display: disp('Unipolar\nBarker Code')
  Frame Conversion : FrameConversion  OutFrame=Sample-based
  Matrix Concatenate : Concatenate  NumInputs=3  Mode=Multidimensional array
  Random Interleaver : commblkintrlv2/Random Interleaver  N=qpsktxrx.DataLength  seed=12345
      settings: SourceProductName=Communications System Toolbox  SourceProductBaseCode=CM
  Repeat : dspsigops/Repeat  N=4  InputProcessing=Columns as channels (frame based)  RateOptions=Enforce single-rate processing  ic=0  mode=Unused parameter value
      settings: SourceProductName=DSP System Toolbox
  Signal From Workspace : dspsrcs4/Signal From Workspace  X=qpsktxrx.sBit2  Ts=-1  nsamps=qpsktxrx.DataLength  OutputAfterFinalValue=Cyclic repetition  ignoreOrWarnInputAndFrameLengths=off  OutputFrames=on
  Out : Outport
  wires:
  Frame Conversion/1 -> Random Interleaver/1
  Repeat/1 -> Matrix Concatenate/2, Matrix Concatenate/1
  Signal From Workspace/1 -> Frame Conversion/1
  Matrix Concatenate/1 -> Out/1
  Barker Code SS/1(Out) -> Repeat/1
  Random Interleaver/1 -> Matrix Concatenate/3

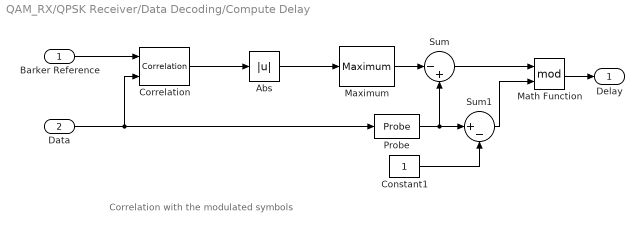
== system QAM_RX/QPSK Receiver/Data Decoding/Compute Delay ==
  note: Correlation with the modulated symbols
  Barker Reference : Inport
  Data : Inport  Port=2
  Abs : Abs
  Constant1 : Constant  VectorParams1D=off  OutDataTypeStr=Inherit: Inherit via back propagation  FramePeriod=2
  Correlation : dspstat3/Correlation  domain=Time  roundingMode=Floor  overflowMode=off  accumDataTypeStr=Inherit: Same as product output  accumLastDataTypeStr=Inherit: Same as product output  outputDataTypeStr=Inherit: Same as accumulator  outputMin=[]  outputMax=[]  outputLastDataTypeStr=Inherit: Same as accumulator
      settings: SourceProductName=DSP System Toolbox  SourceProductBaseCode=DS
  Math Function : Math  Operator=mod  SaturateOnIntegerOverflow=on
  Maximum : dspstat3/Maximum  operation=maximum  fcn=Index  indexBase=One  operateOver=Each column  Dimension=1  InputProcessing=Columns as channels (frame based)  reset=None  roiEnable=off  roiType=Rectangles  roiPortion=Entire ROI  roiOutput=Individual statistics for each ROI  roiFlag=off  roundingMode=Floor  overflowMode=off  accumDataTypeStr=Inherit: Same as product output  accumLastDataTypeStr=Inherit: Same as product output
  Probe : Probe  ProbeSampleTime=off  ProbeComplexSignal=off
  Sum : Sum  Inputs=|-+  SaturateOnIntegerOverflow=on  InputSameDT=on  OutDataTypeStr=Inherit: Same as first input
  Sum1 : Sum  Inputs=|+-  SaturateOnIntegerOverflow=on  InputSameDT=on  OutDataTypeStr=Inherit: Same as first input
  Delay : Outport
  wires:
  Abs/1 -> Maximum/1
  Constant1/1 -> Sum1/2
  Sum1/1 -> Math Function/2
  Math Function/1 -> Delay/1
  Sum/1 -> Math Function/1
  Probe/1 -> Sum1/1, Sum/2
  Correlation/1 -> Abs/1
  Maximum/1 -> Sum/1
  Barker Reference/1 -> Correlation/1
  Data/1 -> Correlation/2, Probe/1

== system QAM_RX/QPSK Receiver/Data Decoding/Descrambling ==
  In : Inport
  Random Deinterleaver : commblkintrlv2/Random Deinterleaver  N=qpsktxrx.DataLength  seed=12345
      settings: SourceProductName=Communications System Toolbox  SourceProductBaseCode=CM
  Selector : Selector  IndexOptions=Index vector (dialog)  Indices=[qpsktxrx.BarkerLength*log2(qpsktxrx.M)+1:qpsktxrx.FrameSize*log2(qpsktxrx.M)]  OutputSizes=1
  Signal To Workspace : SignalToWorkspace  Commented=on  VariableName=after_deinterleaver
      settings: CopyFcn=dspblkcopystw(gcbh);
  Signal To Workspace1 : SignalToWorkspace  Commented=on  VariableName=before_deinterleaver
      settings: CopyFcn=dspblkcopystw(gcbh);
  Signal To Workspace2 : SignalToWorkspace  Commented=on  VariableName=received_complete
      settings: CopyFcn=dspblkcopystw(gcbh);
  Out : Outport
  wires:
  Selector/1 -> Random Deinterleaver/1, Signal To Workspace1/1
  In/1 -> Signal To Workspace2/1, Selector/1
  Random Deinterleaver/1 -> Out/1, Signal To Workspace/1

== system QAM_RX/QPSK Receiver/Data Decoding/Phase Ambiguity Correction & Demodulation ==
  note: Phase Ambiguity Resolution
      | and Demodulation
  Phase : Inport
  Data : Inport  Port=2
  Complex Phase Shift : commutil2/Complex Phase Shift
      settings: SourceProductName=Communications System Toolbox  SourceProductBaseCode=CM
  Corrected Symbols : ConstellationDiagram  Tag=ScatterPlot
  Gain : Gain  Gain=-1  OutDataTypeStr=Inherit: Same as input
  MLSE Equalizer : commeq2/MLSE Equalizer  Commented=on  specchan=Dialog  chancoeff=[1 0.7 0.5 0.3]'  constpts=[1+j -1+j -1-j 1-j 3+j -3+j -3-j 3-j 3+3j -3+3j -3-3j 3-3j 1+3j -1+3j -1-3j 1-3j]  tbdepth=21  opmode=Reset every frame  enpreamble=off  preamble=[0 3 2 1]  enpostamble=off  postamble=[0 2 3 1]  numsamp=1  reset=off
      settings: SourceProductName=Communications System Toolbox  SourceProductBaseCode=CM
  Probe2 : Probe  ProbeSampleTime=off  ProbeComplexSignal=off
  Rectangular QAM Demodulator Baseband : commdigbbndam3/Rectangular QAM Demodulator Baseband  M=16  OutType=Bit  DecType=Hard decision  VarSource=Dialog  Variance=1  Dec=Gray  Mapping=[0:15]  PowType=Min. distance between symbols  MinDist=2  AvgPow=1  PeakPow=1  Ph=0  outDtype1=Inherit via internal rule  outDtype2=Inherit via internal rule  derotateFactorWordLen=16  derotateFactorDataTypeStr=Inherit: Same word length as input  derotateFactorLastDataTypeStr=Inherit: Same word length as input  denormFactorWordLen=16  denormFactorDataTypeStr=Inherit: Same word length as input  denormFactorLastDataTypeStr=Inherit: Same word length as input  prodOutWordLen=32  prodOutOverflowMode=Wrap  prodOutRoundingMode=Floor  prodOutOvFlMode=off  prodOutOvFlModeLastStrValue=off  sumWordLen=32
  Signal To Workspace2 : SignalToWorkspace  Commented=on  VariableName=after_phase_ambiguity
      settings: CopyFcn=dspblkcopystw(gcbh);
  Out : Outport
  wires:
  Phase/1 -> Gain/1
  Rectangular QAM Demodulator Baseband/1 -> Out/1
  Gain/1 -> Complex Phase Shift/2
  Data/1 -> Complex Phase Shift/1
  Complex Phase Shift/1 -> Rectangular QAM Demodulator Baseband/1, Corrected Symbols/1, Signal To Workspace2/1, Probe2/1

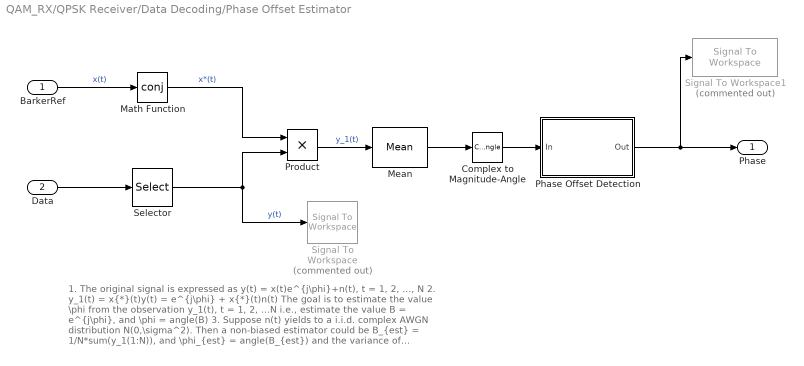
== system QAM_RX/QPSK Receiver/Data Decoding/Phase Offset Estimator ==
  note: 1. The original signal is expressed as y(t) = x(t)e^{j\phi}+n(t), t = 1, 2, ..., N
      | 2. y_1(t) = x{*}(t)y(t) = e^{j\phi} + x{*}(t)n(t)
      | The goal is to estimate the value \phi from the observation y_1(t), t = 1, 2, ...N
      | i.e., estimate the value B = e^{j\phi}, and \phi = angle(B)
      | 3. Suppose n(t) yields to a i.i.d. complex AWGN distribution N(0,\sigma^2).
      | Then a non-biased estimator could be
      | B_{est} = 1/N*sum(y_1(1:N)), and \phi_{est} = angle(B_{est})
      | and the variance of B_{est} is \sigma^2/N
  BarkerRef : Inport
  Data : Inport  Port=2
  Complex to Magnitude-Angle : ComplexToMagnitudeAngle  Output=Angle
  Math Function : Math  Operator=conj  SaturateOnIntegerOverflow=on
  Mean : dspstat3/Mean  run=off  InputProcessing=Columns as channels (frame based)  reset_popup=None  directionMode=Each column  dimension=1  roiEnable=off  roiType=Rectangles  roiPortion=Entire ROI  roiOutput=Individual statistics for each ROI  roiFlag=off  roundingMode=Floor  overflowMode=off  outputDataTypeStr=Inherit: Same as accumulator  outputMin=[]  outputMax=[]  outputLastDataTypeStr=Inherit: Same as accumulator
  Phase Offset Detection : MATLAB Function  TreatAsAtomicUnit=on
  Product : Product  RndMeth=Zero
  Selector : Selector  IndexOptions=Index vector (dialog)  Indices=[1:26]  OutputSizes=1
  Signal To Workspace : SignalToWorkspace  Commented=on  VariableName=received_Barker
      settings: CopyFcn=dspblkcopystw(gcbh);  Save2DSignal=3-D array (concatenate along third dimension)
  Signal To Workspace1 : SignalToWorkspace  Commented=on  VariableName=Phase_lock_error
      settings: CopyFcn=dspblkcopystw(gcbh);  Save2DSignal=3-D array (concatenate along third dimension)
  Phase : Outport
  wires:
  Data/1 -> Selector/1
  BarkerRef/1 -> Math Function/1  "x(t)"
  Selector/1 -> Product/2, Signal To Workspace/1  "y(t)"
  Math Function/1 -> Product/1  "x*(t)"
  Product/1 -> Mean/1  "y_1(t)"
  Mean/1 -> Complex to Magnitude-Angle/1
  Complex to Magnitude-Angle/1 -> Phase Offset Detection/1(In)
  Phase Offset Detection/1(Out) -> Phase/1, Signal To Workspace1/1

== system QAM_RX/QPSK Receiver/Fine Frequency Compensation/DDS ==
  note: The digital filter acts as a pure integrator
  In : Inport
  Digital Filter : dspobslib/Digital Filter  TypePopup=IIR (poles & zeros)  IIRFiltStruct=Direct form II transposed  AllPoleFiltStruct=Direct form  FIRFiltStruct=Direct form  CoeffSource=Specify via dialog  NumCoeffs=[0 1]  DenCoeffs=[1 -1]  BiQuadCoeffs=[1 0.3 0.4 1 0.1 0.2]  LatticeCoeffs=[0.2 0.4]  denIgnore=on  FiltPerSampPopup=One filter per frame  IC=0  ICnum=0  ICden=0  roundingMode=Floor  overflowMode=off  ScaleValues=1  scaleValueFracLength=14  stageInFracLength=15  stageOutFracLength=15  FilterSource=Specify via dialog  dfiltObjectName=dfilt.dffir([1 2 1])  InputProcessing=Columns as channels (frame based)
      settings: SourceProductName=DSP System Toolbox  SourceProductBaseCode=DS
  Gain : Gain  Gain=-1*qpsktxrx.PhaseRecoveryGain
  Phase : Outport
  wires:
  Digital Filter/1 -> Gain/1
  In/1 -> Digital Filter/1
  Gain/1 -> Phase/1

== system QAM_RX/QPSK Receiver/Fine Frequency Compensation/Loop Filter ==
  note: Proportional-plus-Integrator Loop Filter,
      | Infinite DC Response to guarantee convergence
  e : Inport
  Digital Filter : dspobslib/Digital Filter  TypePopup=IIR (poles & zeros)  IIRFiltStruct=Direct form II transposed  AllPoleFiltStruct=Direct form  FIRFiltStruct=Direct form  CoeffSource=Specify via dialog  NumCoeffs=[1 0]  DenCoeffs=[1 -1]  BiQuadCoeffs=[1 0.3 0.4 1 0.1 0.2]  LatticeCoeffs=[0.2 0.4]  denIgnore=on  FiltPerSampPopup=One filter per frame  IC=0  ICnum=0  ICden=0  roundingMode=Floor  overflowMode=off  ScaleValues=1  scaleValueFracLength=14  stageInFracLength=15  stageOutFracLength=15  FilterSource=Specify via dialog  dfiltObjectName=dfilt.dffir([1 2 1])  InputProcessing=Columns as channels (frame based)
      settings: SourceProductName=DSP System Toolbox  SourceProductBaseCode=DS
  K1 : Gain  Gain=K1
  K2 : Gain  Gain=K2
  Sum2 : Sum  SaturateOnIntegerOverflow=on  InputSameDT=on  OutDataTypeStr=Inherit: Same as first input
  v : Outport
  wires:
  K2/1 -> Digital Filter/1
  Digital Filter/1 -> Sum2/2
  Sum2/1 -> v/1
  e/1 -> K2/1, K1/1
  K1/1 -> Sum2/1

== system QAM_RX/QPSK Receiver/Timing Recovery/Enabled Wire ==
  In : Inport
  Enable : EnablePort
  Out : Outport
  wires:
  In/1 -> Out/1

== system QAM_RX/QPSK Receiver/Timing Recovery/Modified Buffer ==
  Data : Inport
  Clk : Inport  Port=2
  Frame Conversion : FrameConversion  OutFrame=Sample-based
  Logical Operator : Logic  AllPortsSameDT=off  OutDataTypeStr=boolean
  Modified Buffer : Subsystem
  DataOut : Outport
  DataValid : Outport  Port=2
  wires:
  Data/1 -> Modified Buffer/1(In)
  Modified Buffer/1(DataOut) -> Frame Conversion/1
  Modified Buffer/2(DataValid) -> Logical Operator/1
  Logical Operator/1 -> DataValid/1
  Frame Conversion/1 -> DataOut/1
  Clk/1 -> Modified Buffer/Enable, Logical Operator/2
